simulink model "Ejercicio_Teorica_Simulink_1"  (R2023b)
settings: Solver=VariableStepAuto  StartTime=0.0  StopTime=10.0  RelTol=1e-3
undefined symbols (not defined in the file or in its folder): A, B, C, K
settings Model: Creator=juanj  LastModifiedBy=juanj

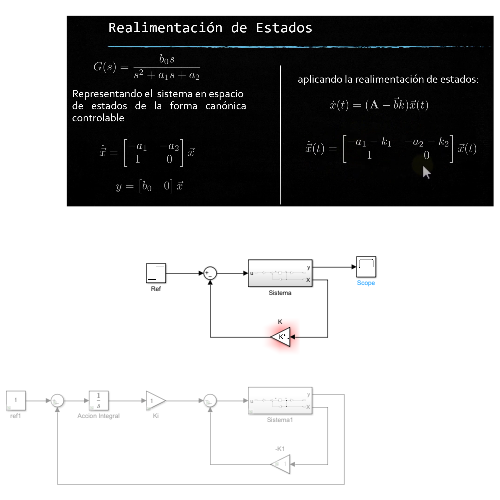
[thumbnail: Simulink's stored preview of the top-level diagram]
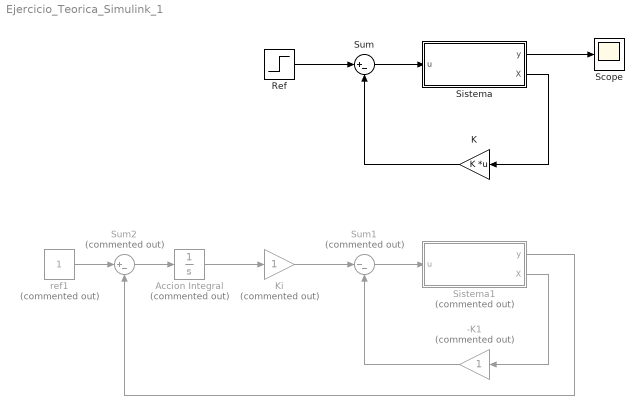
== system Ejercicio_Teorica_Simulink_1 ==
  -K1 : Gain  Commented=on
  Accion Integral : Integrator  Commented=on
  K : Gain  Gain=K  Multiplication=Matrix(K*u)
  Ki : Gain  Commented=on
  Ref : Step  Time=0  SampleTime=0
  Scope : Scope
  Sistema : Subsystem
  Sistema1 : Subsystem  Commented=on
  Sum : Sum  Inputs=|+-
  Sum1 : Sum  Commented=on  Inputs=|--
  Sum2 : Sum  Commented=on  Inputs=|+-
  ref1 : Constant  Commented=on
  wires:
  Sistema/2(X) -> K/1
  Sum/1 -> Sistema/1(u)
  K/1 -> Sum/2
  Sum1/1 -> Sistema1/1(u)
  -K1/1 -> Sum1/2
  Sistema1/2(X) -> -K1/1
  Ki/1 -> Sum1/1
  Accion Integral/1 -> Ki/1
  ref1/1 -> Sum2/1
  Sum2/1 -> Accion Integral/1
  Sistema1/1(y) -> Sum2/2
  Sistema/1(y) -> Scope/1
  Ref/1 -> Sum/1

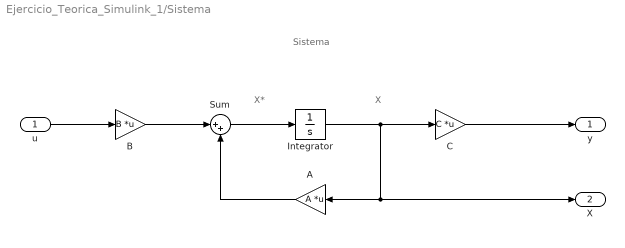
== system Ejercicio_Teorica_Simulink_1/Sistema ==
  note: Sistema
  note: X*
  note: X
  u : Inport
  A : Gain  Gain=A  Multiplication=Matrix(K*u)
  B : Gain  Gain=B  Multiplication=Matrix(K*u)
  C : Gain  Gain=C  Multiplication=Matrix(K*u)
  Integrator : Integrator
  Sum : Sum  Inputs=|++
  y : Outport
  X : Outport  Port=2
  wires:
  u/1 -> B/1
  A/1 -> Sum/2
  Sum/1 -> Integrator/1
  C/1 -> y/1
  B/1 -> Sum/1
  Integrator/1 -> X/1, A/1, C/1

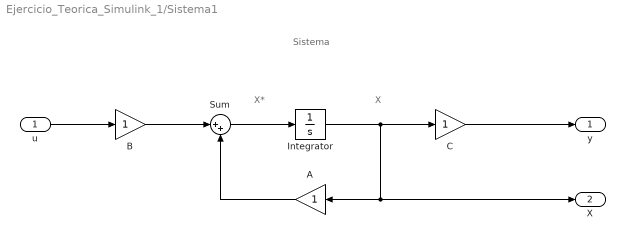
== system Ejercicio_Teorica_Simulink_1/Sistema1 ==
  note: Sistema
  note: X*
  note: X
  u : Inport
  A : Gain
  B : Gain
  C : Gain
  Integrator : Integrator
  Sum : Sum  Inputs=|++
  y : Outport
  X : Outport  Port=2
  wires:
  u/1 -> B/1
  A/1 -> Sum/2
  Sum/1 -> Integrator/1
  C/1 -> y/1
  B/1 -> Sum/1
  Integrator/1 -> X/1, A/1, C/1
